simulink model "Fig357"  (R2014b)
settings: Solver=ode3  StartTime=0.0  StopTime=10.005  FixedStep=2e-6  RelTol=1e-5
libraries: commfilt2 x2, commutil2 x1, commchan3 x1, commsink2 x1, commrandsrc2 x1
settings Model: Creator=Dennis Silage  LastModifiedBy=Silage
settings DataIOCC: SignalLoggingSaveFormat=ModelDataLogs
settings OptimizationCC: ExpressionDepthLimit=2147483647  InitFltsAndDblsToZero=on
settings DebuggingCC: UnderspecifiedInitializationDetection=Classic  MergeDetectMultiDrivingBlocksExec=none  SolverPrmCheckMsg=none  FcnCallInpInsideContextMsg=UseLocalSettings  StateNameClashWarn=warning
settings GRTTargetCC: CombineOutputUpdateFcns=off  GRTInterface=on

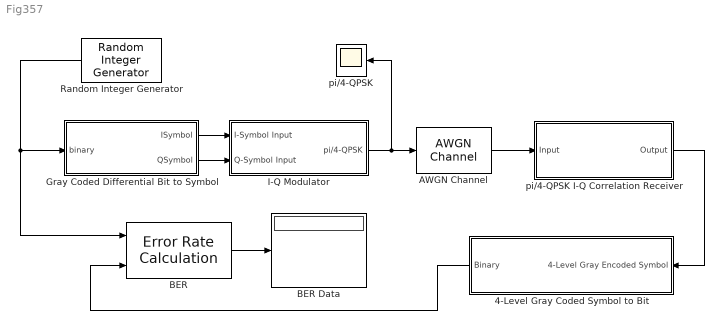
== system Fig357 ==
  4-Level Gray Coded Symbol to Bit : Subsystem
  AWGN Channel : commchan3/AWGN Channel  InputProcessing=Inherited (this choice will be removed - see release notes)  seed=randseed  noiseMode="Signal to noise ratio  (Eb/No)"  EbNodB=50  EsNodB=20  SNRdB=10  bitsPerSym=2  Ps=12.5  Tsym=2e-3  variance=0
  BER : commsink2/Error Rate Calculation  N=6  st_delay=0  cp_mode=Entire frame  subframe=[]  PMode=Port  WsName=ErrorVec  RsMode2=off  stop=off  numErr=100  maxBits=1e6
  BER Data : Display
  Gray Coded Differential Bit to Symbol : MATLAB Function  TreatAsAtomicUnit=on
  I-Q Modulator : Subsystem
  Random Integer Generator : commrandsrc2/Random Integer Generator  mul=2  seed=59  Ts=1e-3  frameBased=off  sampPerFrame=1  orient=off  outDataType=double
  pi/4-QPSK : Scope
      settings: TimeRange=0.005  YMin=-10  YMax=10  MaxDataPoints=8001
  pi/4-QPSK I-Q Correlation Receiver : Subsystem
  wires:
  BER/1 -> BER Data/1
  I-Q Modulator/1(pi/4-QPSK) -> AWGN Channel/1, pi/4-QPSK/1
  AWGN Channel/1 -> pi/4-QPSK I-Q Correlation Receiver/1(Input)
  pi/4-QPSK I-Q Correlation Receiver/1(Output) -> 4-Level Gray Coded Symbol to Bit/1(4-Level Gray Encoded Symbol)
  4-Level Gray Coded Symbol to Bit/1(Binary) -> BER/2
  Gray Coded Differential Bit to Symbol/2(QSymbol) -> I-Q Modulator/2(Q-Symbol Input)
  Gray Coded Differential Bit to Symbol/1(ISymbol) -> I-Q Modulator/1(I-Symbol Input)
  Random Integer Generator/1 -> Gray Coded Differential Bit to Symbol/1(binary), BER/1

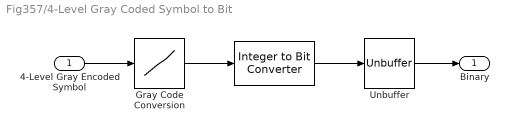
== system Fig357/4-Level Gray Coded Symbol to Bit ==
  4-Level Gray Encoded Symbol : Inport
  " " : commutil2/Integer to Bit Converter  nbits=2  signedInputValues=Unsigned  bitOrder=MSB first  outDtype=double
  Gray Code Conversion : Lookup_n-D  NumberOfTableDimensions=1  BreakpointsForDimension1=[0 1 2 3]  Table=[0 1 3 2]  InternalRulePriority=Speed  RndMeth=Simplest  InputSameDT=on
  Unbuffer : Unbuffer  SampleBasedProcessing=Same as frame based
  Binary : Outport
  wires:
  " "/1 -> Unbuffer/1
  4-Level Gray Encoded Symbol/1 -> Gray Code Conversion/1
  Unbuffer/1 -> Binary/1
  Gray Code Conversion/1 -> " "/1

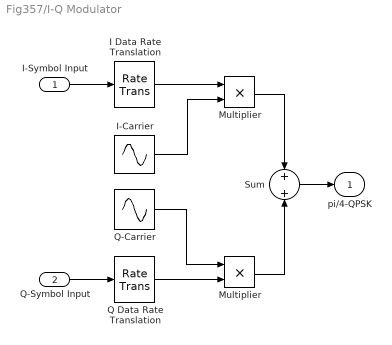
== system Fig357/I-Q Modulator ==
  I-Symbol Input : Inport
  Q-Symbol Input : Inport  Port=2
  " Multiplier " : Product  RndMeth=Zero
  I Data Rate Translation : RateTransition  Integrity=off  Deterministic=off  OutPortSampleTime=2e-6
  I-Carrier : Sin  Amplitude=5  Frequency=40000*pi  Phase=pi/2  SampleTime=2e-6  VectorParams1D=off
  Multiplier : Product  RndMeth=Zero
  Q Data Rate Translation : RateTransition  Integrity=off  OutPortSampleTime=2e-6
  Q-Carrier : Sin  Amplitude=5  Frequency=40000*pi  SampleTime=2e-6  VectorParams1D=off
  Sum : Sum
  pi/4-QPSK : Outport
  wires:
  I Data Rate Translation/1 -> Multiplier/1
  Q Data Rate Translation/1 -> " Multiplier "/2
  I-Carrier/1 -> Multiplier/2
  Q-Carrier/1 -> " Multiplier "/1
  Multiplier/1 -> Sum/1
  " Multiplier "/1 -> Sum/2
  Sum/1 -> pi/4-QPSK/1
  I-Symbol Input/1 -> I Data Rate Translation/1
  Q-Symbol Input/1 -> Q Data Rate Translation/1

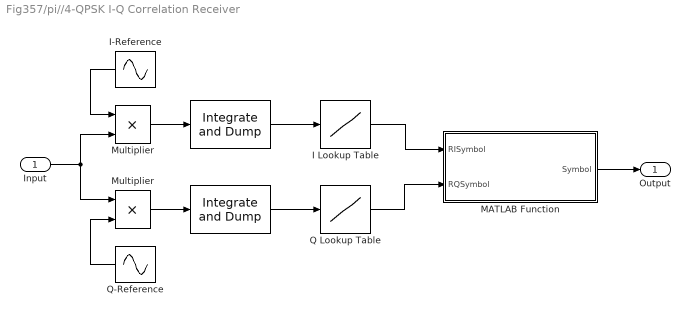
== system Fig357/pi//4-QPSK I-Q Correlation Receiver ==
  Input : Inport
  " " : commfilt2/Integrate and Dump  obssamples=1000  offsetsamples=500  nodump=off  roundingMode=Floor  overflowMode=off
  "  " : commfilt2/Integrate and Dump  obssamples=1000  offsetsamples=500  nodump=off  roundingMode=Floor  overflowMode=off
  I Lookup Table : Lookup_n-D  NumberOfTableDimensions=1  BreakpointsForDimension1=[-12500 -8838.8 0 8838.8 12500]  Table=[-1 -0.70705 0 0.70705 1]  InterpMethod=Nearest  InternalRulePriority=Speed  RndMeth=Simplest  InputSameDT=on
  I-Reference : Sin  Amplitude=5  Frequency=40000*pi  Phase=pi/2  SampleTime=2e-6
  MATLAB Function : MATLAB Function  TreatAsAtomicUnit=on
  Multiplier : Product  RndMeth=Zero
  "Multiplier " : Product  RndMeth=Zero
  Q Lookup Table : Lookup_n-D  NumberOfTableDimensions=1  BreakpointsForDimension1=[-12500 -8838.8 0 8838.8 12500]  Table=[-1 -0.70705 0 0.70705 1]  InterpMethod=Nearest  InternalRulePriority=Speed  RndMeth=Simplest  InputSameDT=on
  Q-Reference : Sin  Amplitude=5  Frequency=40000*pi  SampleTime=2e-6
  Output : Outport
  wires:
  "Multiplier "/1 -> " "/1
  Multiplier/1 -> "  "/1
  I-Reference/1 -> "Multiplier "/1
  Q-Reference/1 -> Multiplier/2
  Input/1 -> "Multiplier "/2, Multiplier/1
  MATLAB Function/1(Symbol) -> Output/1
  " "/1 -> I Lookup Table/1
  "  "/1 -> Q Lookup Table/1
  I Lookup Table/1 -> MATLAB Function/1(RISymbol)
  Q Lookup Table/1 -> MATLAB Function/2(RQSymbol)

== matlab function Fig357/Gray Coded Differential Bit to Symbol ==
  data: binary input; ISymbol output; QSymbol output
function [ISymbol, QSymbol]  = fcn(binary)
%#codegen
persistent flag dIbit dISymbol dQSymbol

if isempty(flag)
    flag = 0;
    dISymbol = 1;       %initial values  
    dQSymbol = 0;
    dIbit = 0;
end

if (flag == 0)          %MSB
    ISymbol = dISymbol;
    QSymbol = dQSymbol;
    dIbit = binary;
    flag = 1;
else
    if (dIbit == 1)     %Gray codingo using LSB
        if (binary == 0)
            binary = 1;
        else
            binary = 0;
        end
    end
    Qbit = 2*(binary - 0.5);
    Ibit = 2*(dIbit - 0.5);
    ISymbol = (dISymbol*Ibit - dQSymbol*Qbit)/1.4142135;
    QSymbol = (dISymbol*Qbit + dQSymbol*Ibit)/1.4142135;
    dISymbol = ISymbol;
    dQSymbol = QSymbol;
    flag = 0;
end

end

== matlab function Fig357/pi//4-QPSK I-Q Correlation Receiver/MATLAB Function ==
  data: RISymbol input; Symbol output; RQSymbol input
function Symbol  = fcn(RISymbol, RQSymbol)
%#codegen
persistent dRISymbol dRQSymbol

if isempty(dRISymbol)
    dRISymbol = 0;
    dRQSymbol = 0;
    Symbol = 0;
end

    if ((RQSymbol*dRQSymbol + RISymbol*dRISymbol)>0)
        MSB = 1;
    else
        MSB = 0;
    end
    if ((dRISymbol*RQSymbol - RISymbol*dRQSymbol)>0)
        LSB = 1;
    else
        LSB = 0;
    end
    dRISymbol = RISymbol;
    dRQSymbol = RQSymbol;    
    Symbol = 2*MSB + LSB;
    
end
